simulink model "qtest2"  (Simulink 7.0)
settings: Solver=ode5  StartTime=0.0  StopTime=stop_time  FixedStep=step_size  RelTol=1e-3
libraries: qlib x3
Description:
  | Unit Test for Quaternion Library: Integration block
  | 
  | Copyright (c) 2001-2009, Jay A. St. Pierre.  All rights reserved.
settings Model: Creator=stpierre  LastModifiedBy=stpierre  ExtModeTrigMode=oneshot  ExtModeArmWhenConnect=off  ExtModeAutoUpdateStatusClock=off
settings DataIOCC: Decimation=decimation  LimitDataPoints=off  SaveOutput=off
settings OptimizationCC: BlockReduction=off  BooleanDataType=off
settings DebuggingCC: SaveWithParameterizedLinksMsg=none  SignalResolutionControl=TryResolveAllWithWarning  SolverPrmCheckMsg=none  MultiTaskDSMMsg=warning  MultiTaskCondExecSysMsg=none
settings HardwareCC: TargetUnknown=on
settings RTWCC: IncludeERTFirstTime=on

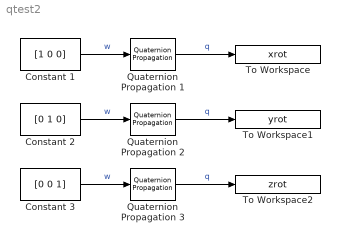
== system qtest2 ==
  Constant 1 : Constant  Value=[1 0 0]
  Constant 2 : Constant  Value=[0 1 0]
  Constant 3 : Constant  Value=[0 0 1]
  Quaternion Propagation 1 : qlib/Quaternion Propagation  SystemSampleTime=-1  q0=[0 0 0 1]
  Quaternion Propagation 2 : qlib/Quaternion Propagation  SystemSampleTime=-1  q0=[0 0 0 1]
  Quaternion Propagation 3 : qlib/Quaternion Propagation  SystemSampleTime=-1  q0=[0 0 0 1]
  To Workspace : ToWorkspace  VariableName=xrot  SampleTime=-1  SaveFormat=Array
      settings: MaxDataPoints=10000  Decimation=decimation
  To Workspace1 : ToWorkspace  VariableName=yrot  SampleTime=-1  SaveFormat=Array
      settings: MaxDataPoints=10000  Decimation=decimation
  To Workspace2 : ToWorkspace  VariableName=zrot  SampleTime=-1  SaveFormat=Array
      settings: MaxDataPoints=10000  Decimation=decimation
  wires:
  Constant 1/1 -> Quaternion Propagation 1/1  "w"
  Quaternion Propagation 1/1 -> To Workspace/1  "q"
  Constant 2/1 -> Quaternion Propagation 2/1  "w"
  Quaternion Propagation 2/1 -> To Workspace1/1  "q"
  Constant 3/1 -> Quaternion Propagation 3/1  "w"
  Quaternion Propagation 3/1 -> To Workspace2/1  "q"
